simulink model "model_tracking"  (R2015a)
settings: Solver=ode45  StartTime=0.0  StopTime=Tend  RelTol=1e-3
values from neighbouring files (symbols this model uses):
  A = [-31.31 0 -2.833e4 2; 0 -10.25 8001 0; 1 -1 0 0; 0 0 0 -100]    [Copy_of_UIE_tracking_main.m]    (also in UIE_main.m = [0 0 1 0; 0 0 0 1; -3 1 -0.4 0.1; 1 -1 0.1 -0.1]; UIE_tracking_main.m = [0 0 1 0; 0 0 0 1; -3 1 -0.4 0.1; 1 -1 0.1 -0.1])
  Af = [-100 0; 0 -100]    [Copy_of_UIE_tracking_main.m]    (also in UIE_main.m; UIE_tracking_main.m)
  B = [28.06 0 0 1; 0 28.06 0 1]'    [Copy_of_UIE_tracking_main.m]    (also in UIE_main.m = [0 0; 0 0; 1 0; 0 1]; UIE_tracking_main.m = [0 0; 0 0; 1 0; 0 1])
  Bd = B    [Copy_of_UIE_tracking_main.m]    (also in UIE_main.m = [0 0 0; 0 0 0; 1 0.5 0.75; 0.5 1 0.75]; UIE_tracking_main.m)
  Bf = [8 0; 0 8]    [Copy_of_UIE_tracking_main.m]    (also in UIE_main.m; UIE_tracking_main.m)
  C = [1 0 0 0;1 0 30 0]    [Copy_of_UIE_tracking_main.m]    (also in UIE_main.m = [1 0 0 0; 0 1 0 0]; UIE_tracking_main.m = [1 0 0 0; 0 1 0 0])
  Cf = [12.5 0; 0 12.5]    [Copy_of_UIE_tracking_main.m]    (also in UIE_main.m; UIE_tracking_main.m)
  Ec = -inv(Rc)*B'*inv(A - B*Kc)'*C'*Qc    [Copy_of_UIE_tracking_main.m]    (also in UIE_main.m; UIE_tracking_main.m)
  Kc = lqr(A + Hc*eye(n), B, C'*Qc*C, Rc)    [Copy_of_UIE_tracking_main.m]    (also in UIE_main.m; UIE_tracking_main.m)
  Kd = pinv(B)*Lt    [Copy_of_UIE_tracking_main.m]    (also in UIE_main.m; UIE_tracking_main.m)
  L = lqr(A'+H*eye(n), C', Qo, Ro)'    [Copy_of_UIE_tracking_main.m]    (also in UIE_main.m; UIE_tracking_main.m)
  Tf = 1e-3    (= 0.001)    [Copy_of_UIE_tracking_main.m]    (also in UIE_main.m; UIE_tracking_main.m)
  x_ini = [0 0 0 0]    [Copy_of_UIE_tracking_main.m]    (also in UIE_main.m = [0 1 0 0]; UIE_tracking_main.m)
  xo_ini = [0 0 0 0]    [Copy_of_UIE_tracking_main.m]    (also in UIE_main.m = [0 1 0 0]; UIE_tracking_main.m)
settings Model: CovSFcnEnable=off  Creator=123  LastModifiedBy=Elca
settings DebuggingCC: SolverPrmCheckMsg=warning  UnconnectedInputMsg=none  UnconnectedOutputMsg=none

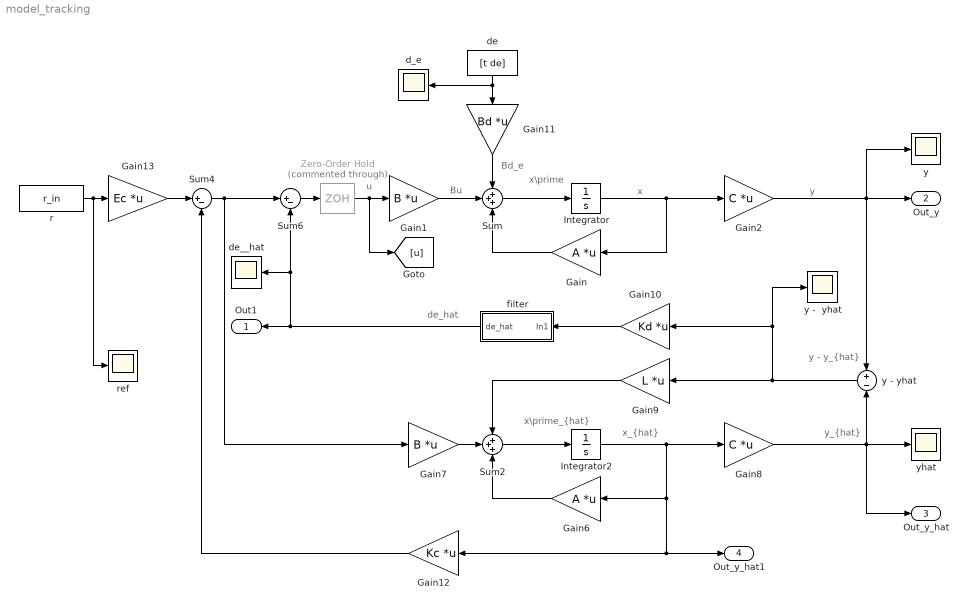
== system model_tracking ==
  note: de_hat
  note: Bd_e
  note: Bu
  note: y - y_{hat}
  note: x\prime
  note: x\prime_{hat}
  note: x_{hat}
  note: y_{hat}
  note: x
  note: y
  note: u
  Gain : Gain  Gain=A  Multiplication=Matrix(K*u)
  Gain1 : Gain  Gain=B  Multiplication=Matrix(K*u)
  Gain10 : Gain  Gain=Kd  Multiplication=Matrix(K*u)
  Gain11 : Gain  Gain=Bd  Multiplication=Matrix(K*u)
  Gain12 : Gain  Gain=Kc  Multiplication=Matrix(K*u)
  Gain13 : Gain  Gain=Ec  Multiplication=Matrix(K*u)
  Gain2 : Gain  Gain=C  Multiplication=Matrix(K*u)
  Gain6 : Gain  Gain=A  Multiplication=Matrix(K*u)
  Gain7 : Gain  Gain=B  Multiplication=Matrix(K*u)
  Gain8 : Gain  Gain=C  Multiplication=Matrix(K*u)
  Gain9 : Gain  Gain=L  Multiplication=Matrix(K*u)
  Integrator : Integrator  InitialCondition=x_ini
  Integrator2 : Integrator  InitialCondition=xo_ini
  Sum : Sum  Inputs=+++
  Sum2 : Sum  Inputs=+++
  Sum4 : Sum  Inputs=|+-
  Sum6 : Sum  Inputs=|+-
  Zero-Order Hold : ZeroOrderHold  Commented=through  SampleTime=Tf
  d_e : Scope
      settings: TickLabels=on  ShowLegends=on  ScrollMode=on
  de : FromWorkspace  VariableName=[t de]  SampleTime=0
  de__hat : Scope
      settings: TickLabels=on  ShowLegends=on  SaveName=ScopeData2  ScrollMode=on
  filter : Subsystem
  r : FromWorkspace  VariableName=r_in  SampleTime=Tf
  ref : Scope
      settings: TickLabels=on  YMin=0  YMax=550000  SaveName=ScopeData5  ScrollMode=on
  y : Scope
      settings: TickLabels=on  YMin=0  YMax=550000  SaveName=ScopeData4  ScrollMode=on
  y -  yhat : Scope
      settings: TickLabels=on  ShowLegends=on  ScrollMode=on
  y - yhat : Sum  Inputs=+-
  yhat : Scope
      settings: TickLabels=on  ShowLegends=on  SaveName=ScopeData3  ScrollMode=on
  Out1 : Outport
  Out_y : Outport  Port=2
  Out_y_hat : Outport  Port=3
  Out_y_hat1 : Outport  Port=4
  wires:
  Sum/1 -> Integrator/1
  Integrator/1 -> Gain/1, Gain2/1
  Sum2/1 -> Integrator2/1
  Integrator2/1 -> Out_y_hat1/1, Gain12/1, Gain6/1, Gain8/1
  Gain6/1 -> Sum2/3
  Gain7/1 -> Sum2/2
  y - yhat/1 -> Gain9/1, Gain10/1, y -  yhat/1
  Gain9/1 -> Sum2/1
  Gain8/1 -> Out_y_hat/1, y - yhat/2, yhat/1
  Gain2/1 -> y - yhat/1, y/1, Out_y/1
  Sum6/1 -> Zero-Order Hold/1
  de/1 -> Gain11/1, d_e/1
  Gain/1 -> Sum/3
  Gain1/1 -> Sum/2
  Gain12/1 -> Sum4/2
  Sum4/1 -> Gain7/1, Sum6/1
  Gain13/1 -> Sum4/1
  r/1 -> ref/1, Gain13/1
  Zero-Order Hold/1 -> Gain1/1, [u]
  Gain10/1 -> filter/1(In1)
  Gain11/1 -> Sum/1
  filter/1(de_hat) -> Sum6/2, de__hat/1, Out1/1

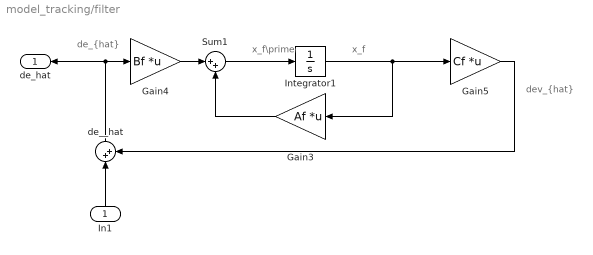
== system model_tracking/filter ==
  note: x_f\prime
  note: x_f
  note: dev_{hat}
  note: de_{hat}
  In1 : Inport
  Gain3 : Gain  Gain=Af  Multiplication=Matrix(K*u)
  Gain4 : Gain  Gain=Bf  Multiplication=Matrix(K*u)
  Gain5 : Gain  Gain=Cf  Multiplication=Matrix(K*u)
  Integrator1 : Integrator
  Sum1 : Sum  Inputs=|++
  de__hat : Sum  Inputs=|++
  de_hat : Outport
  wires:
  Gain4/1 -> Sum1/1
  Sum1/1 -> Integrator1/1
  Integrator1/1 -> Gain3/1, Gain5/1
  Gain3/1 -> Sum1/2
  de__hat/1 -> de_hat/1, Gain4/1
  Gain5/1 -> de__hat/2
  In1/1 -> de__hat/1
